simulink model "precom_dyn_1"  (Simulink 8.5)
settings: Solver=ode45  StartTime=0.0  StopTime=5  FixedStep=.001  RelTol=1e-3
undefined symbols (not defined in the file or in its folder): A, B, C, F, K
libraries: cstblocks x3
settings Model: Creator=user  LastModifiedBy=glebret
settings SolverCC: ZeroCrossControl=EnableAll  PositivePriorityOrder=on
settings DataIOCC: LimitDataPoints=off
settings OptimizationCC: BooleanDataType=off  ExpressionDepthLimit=128  InitFltsAndDblsToZero=on
settings DebuggingCC: SaveWithParameterizedLinksMsg=none  SignalResolutionControl=TryResolveAllWithWarning  MultiTaskDSMMsg=warning  MultiTaskCondExecSysMsg=none  FcnCallInpInsideContextMsg=UseLocalSettings  StateNameClashWarn=none
settings HardwareCC: TargetUnknown=on
settings GRTTargetCC: TargetFcnLib=ansi_tfl_tmw.mat

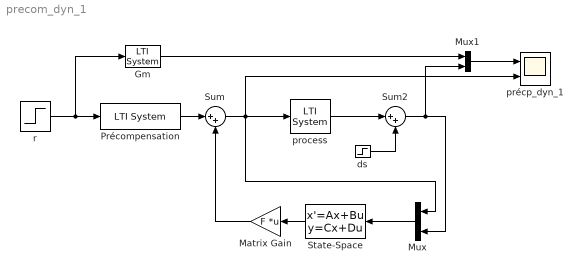
== system precom_dyn_1 ==
  Gm : cstblocks/LTI System  sys=Gm  IC=[]
  Matrix Gain : Gain  Gain=F  Multiplication=Matrix(K*u)  SaturateOnIntegerOverflow=on  OutDataTypeStr=Inherit: Same as input  ParamDataTypeStr=Inherit: Same as input
  Mux : Mux  Inputs=2
  Mux1 : Mux  Inputs=2
  Précompensation : cstblocks/LTI System  sys=precomp_dyn  IC=[]
  State-Space : StateSpace  A=A-K*C  B=[B K]  C=eye(3)  D=zeros(3,2)  X0=0
  Sum : Sum  Inputs=|++  SaturateOnIntegerOverflow=on  InputSameDT=on  OutDataTypeStr=Inherit: Same as first input
  Sum2 : Sum  Inputs=|++  SaturateOnIntegerOverflow=on  InputSameDT=on  OutDataTypeStr=Inherit: Same as first input
  ds : Step  Time=3  SampleTime=0
  process : cstblocks/LTI System  sys=Gp  IC=[]
  précp_dyn_1 : Scope  NumInputPorts=2
      settings: TimeRange=5  YMin=0~-400  YMax=3~200  SaveName=y_dyn_1
  r : Step  SampleTime=0
  wires:
  Mux/1 -> State-Space/1
  State-Space/1 -> Matrix Gain/1
  Matrix Gain/1 -> Sum/2
  Sum/1 -> process/1, précp_dyn_1/2, Mux/1
  Précompensation/1 -> Sum/1
  r/1 -> Précompensation/1, Gm/1
  Mux1/1 -> précp_dyn_1/1
  process/1 -> Sum2/1
  Sum2/1 -> Mux/2, Mux1/2
  ds/1 -> Sum2/2
  Gm/1 -> Mux1/1
